simulink model "Aufgabe8"  (R2016a)
settings: Solver=FixedStepDiscrete  StartTime=0.0  StopTime=inf  RelTol=1e-3
undefined symbols (not defined in the file): gcbh, rcfiltgaincompat, Tbit5_0
libraries: commfilt2 x2, commdigbbndam3 x1, commrandsrc2 x1, NoiseLib_2019 x1
settings Model: Creator=Praktikum  LastModifiedBy=Bornitz
settings DataIOCC: LimitDataPoints=on  SaveFormat=Array
settings OptimizationCC: ExpressionDepthLimit=2147483647  InitFltsAndDblsToZero=on
settings DebuggingCC: SaveWithParameterizedLinksMsg=none  SignalResolutionControl=TryResolveAllWithWarning  SolverPrmCheckMsg=warning  MultiTaskDSMMsg=warning  MultiTaskCondExecSysMsg=none  AllowSymbolicDim=off  StateNameClashWarn=warning  StrictBusMsg=WarnOnBusTreatedAsVector
settings HardwareCC: ProdBitPerPointer=32  ProdLargestAtomicFloat=None  ProdIntDivRoundTo=Undefined  ProdEndianess=Unspecified  ProdWordSize=32  ProdHWDeviceType=32-bit Generic
settings ModelReferenceCC: PropagateSignalLabelsOutOfModel=off
settings SFSimCC: SimParseCustomCode=off
settings GRTTargetCC: TargetFcnLib=ansi_tfl_tmw.mat  CombineOutputUpdateFcns=off  GRTInterface=on
settings ConfigComp: CovModelRefEnable=Off

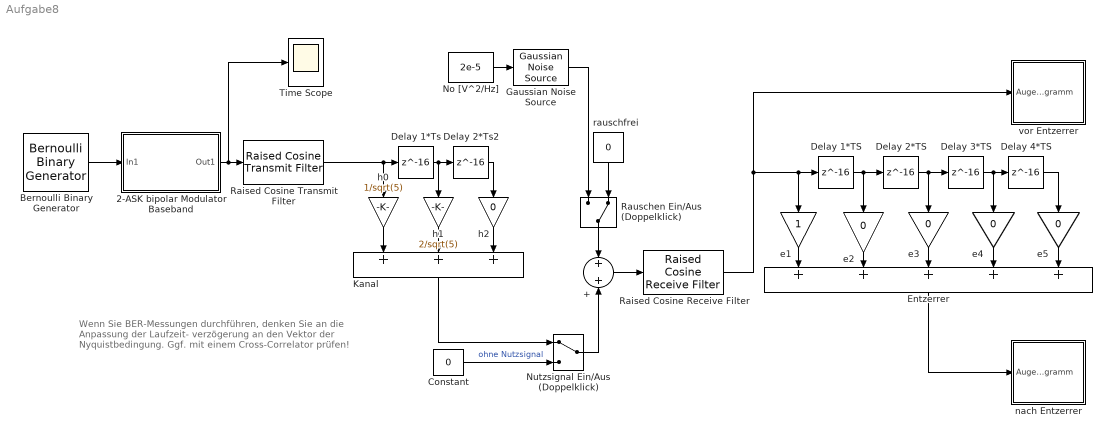
== system Aufgabe8 ==
  note: Wenn Sie BER-Messungen durchführen,
      | denken Sie an die Anpassung der Laufzeit-
      | verzögerung an den Vektor der Nyquistbedingung.
      | Ggf. mit einem Cross-Correlator prüfen!
  " Delay 1*TS" : Delay  DelayLength=16  InitialCondition=0  InputProcessing=Columns as channels (frame based)
  " Delay 1*Ts" : Delay  DelayLength=16  InitialCondition=0  InputProcessing=Columns as channels (frame based)
  " Delay 2*TS" : Delay  DelayLength=16  InitialCondition=0  InputProcessing=Columns as channels (frame based)
  " Delay 2*Ts2" : Delay  DelayLength=16  InitialCondition=0  InputProcessing=Columns as channels (frame based)
  " Delay 3*TS" : Delay  DelayLength=16  InitialCondition=0  InputProcessing=Columns as channels (frame based)
  " Delay 4*TS" : Delay  DelayLength=16  InitialCondition=0  InputProcessing=Columns as channels (frame based)
  + : Sum  SampleTime=Tbit5_0/16
  2-ASK bipolar Modulator Baseband : Subsystem
      mask Display:
      | plot(0,0,100,100,[5+15*[0 1 1 2 2 3] 50 50 50 50+1.5*[[0:.8:10] [10:1.6:20] [20:.8:30]]],[85+8*[1 1 -1 -1 1 1] 85 99 75 85+10*[sin([0:.8:10]*pi*2/5) sin([10:1.6:20]*pi/5) sin([20:.8:30]*pi*2/5)]]);
      | disp('\nGeneral\nASK-Modulator')
  Bernoulli Binary Generator : commrandsrc2/Bernoulli Binary Generator  P=0.5  seed=61  Ts=Tbit5_0  frameBased=off  sampPerFrame=1  orient=off  outDataType=double
  Constant : Constant  Value=0
  Entzerrer : Sum  Inputs=+++++
  Gaussian Noise Source : NoiseLib_2019/Gaussian Noise Source  SystemSampleTime=-1
  Kanal : Sum  Inputs=+++  SampleTime=Tbit5_0/16
  No [V^2/Hz] : Constant  Value=2e-5
  Nutzsignal Ein/Aus (Doppelklick) : ManualSwitch
  Raised Cosine Receive Filter : commfilt2/Raised Cosine Receive Filter  filtType=Square root  R=0.5  filtSpan=2*(4)  N=16  downFactor=1  downOffset=0  filterGain=(0.25)*rcfiltgaincompat(gcbh)  RateOptions=Allow multirate processing  framing=Mute  checkCoeff=off  variableName=rcRxFilt  currentFiltSpan=2*(4)  D=4  inputOffset=0  sampMode=Mute  saveAsFlag=0  rateMode=Downsampling  checkGain=User-specified  launchFVT=off  roundingMode=Floor  overflowMode=off  coeffDataTypeStr=Inherit: Same word length as input  coeffMin=[]  coeffMax=[]  coeffLastDataTypeStr=Inherit: Same word length as input  accumDataTypeStr=Inherit: Same as product output  accumLastDataTypeStr=Inherit: Same as product output  outputDataTypeStr=Inherit: Same as accumulator  outputMin=[]  outputMax=[]  outputLastDataTypeStr=Inherit: Same as accumulator
  Raised Cosine Transmit Filter : commfilt2/Raised Cosine Transmit Filter  filtType=Square root  R=0.5  filtSpan=2*(4)  N=16  filterGain=(4)*rcfiltgaincompat(gcbh)  RateOptions=Allow multirate processing  framing=Mute  checkCoeff=off  variableName=rcTxFilt  checkGain=User-specified  sampMode=Mute  saveAsFlag=0  currentFiltSpan=2*(4)  D=4  launchFVT=off  roundingMode=Floor  overflowMode=off  coeffDataTypeStr=Inherit: Same word length as input  coeffMin=[]  coeffMax=[]  coeffLastDataTypeStr=Inherit: Same word length as input  outputDataTypeStr=Inherit: Same as accumulator  outputMin=[]  outputMax=[]  outputLastDataTypeStr=Inherit: Same as accumulator
  Rauschen Ein/Aus (Doppelklick) : ManualSwitch  CurrentSetting=0
  Time Scope : Scope
  e1 : Gain
  e{2..5} (4 alike) : Gain  Gain=0
  h0 : Gain  Gain=1/sqrt(5)
  h1 : Gain  Gain=2/sqrt(5)
  h2 : Gain  Gain=0
  nach Entzerrer : Subsystem
  rauschfrei : Constant  Value=0
  vor Entzerrer : Subsystem
  wires:
  Bernoulli Binary Generator/1 -> 2-ASK bipolar Modulator Baseband/1(In1)
  +/1 -> Raised Cosine Receive Filter/1
  Constant/1 -> Nutzsignal Ein/Aus (Doppelklick)/2  "ohne Nutzsignal"
  Nutzsignal Ein/Aus (Doppelklick)/1 -> +/2
  e1/1 -> Entzerrer/1
  " Delay 1*TS"/1 -> e2/1, " Delay 2*TS"/1
  e2/1 -> Entzerrer/2
  " Delay 2*TS"/1 -> e3/1, " Delay 3*TS"/1
  e3/1 -> Entzerrer/3
  e4/1 -> Entzerrer/4
  Rauschen Ein/Aus (Doppelklick)/1 -> +/1
  " Delay 3*TS"/1 -> " Delay 4*TS"/1, e4/1
  " Delay 4*TS"/1 -> e5/1
  Raised Cosine Receive Filter/1 -> " Delay 1*TS"/1, e1/1, vor Entzerrer/1(Augendiagramm)
  e5/1 -> Entzerrer/5
  2-ASK bipolar Modulator Baseband/1(Out1) -> Raised Cosine Transmit Filter/1, Time Scope/1
  Gaussian Noise Source/1 -> Rauschen Ein/Aus (Doppelklick)/1
  rauschfrei/1 -> Rauschen Ein/Aus (Doppelklick)/2
  Raised Cosine Transmit Filter/1 -> h0/1, " Delay 1*Ts"/1
  h0/1 -> Kanal/1
  h1/1 -> Kanal/2
  Kanal/1 -> Nutzsignal Ein/Aus (Doppelklick)/1
  " Delay 2*Ts2"/1 -> h2/1
  " Delay 1*Ts"/1 -> " Delay 2*Ts2"/1, h1/1
  h2/1 -> Kanal/3
  No [V^2/Hz]/1 -> Gaussian Noise Source/1
  Entzerrer/1 -> nach Entzerrer/1(Augendiagramm)

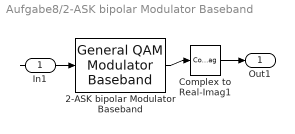
== system Aufgabe8/2-ASK bipolar Modulator Baseband ==
  In1 : Inport
  2-ASK bipolar Modulator Baseband : commdigbbndam3/General QAM Modulator Baseband  SigCon=sig2bp  outDtype=double  outWordLen=16  outUDDataType=sfix(16)  outFracLenMode=Best precision  outFracLen=15  outDataTypeStr=double  outLastDataTypeStr=double
  Complex to Real-Imag1 : ComplexToRealImag  Output=Real
  Out1 : Outport
  wires:
  2-ASK bipolar Modulator Baseband/1 -> Complex to Real-Imag1/1
  In1/1 -> 2-ASK bipolar Modulator Baseband/1
  Complex to Real-Imag1/1 -> Out1/1

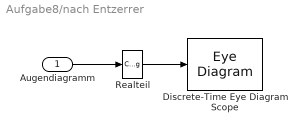
== system Aufgabe8/nach Entzerrer ==
  Augendiagramm : Inport
  Discrete-Time Eye Diagram Scope : EyeDiagram  Tag=EyeDiagram
  Realteil : ComplexToRealImag  Output=Real
  wires:
  Augendiagramm/1 -> Realteil/1
  Realteil/1 -> Discrete-Time Eye Diagram Scope/1

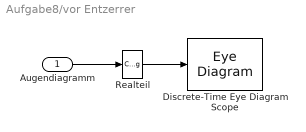
== system Aufgabe8/vor Entzerrer ==
  Augendiagramm : Inport
  Discrete-Time Eye Diagram Scope : EyeDiagram  Tag=EyeDiagram
  Realteil : ComplexToRealImag  Output=Real
  wires:
  Augendiagramm/1 -> Realteil/1
  Realteil/1 -> Discrete-Time Eye Diagram Scope/1
